simulink model "PumpSim"  (R2016b)
settings: Solver=VariableStepAuto  StartTime=0.0  StopTime=10.0  RelTol=1e-3
values from neighbouring files (symbols this model uses):
  A = pi*(0.00635)^2    (= 0.000126676869774)    [PumpParam.m]
  g = 9.8    [MotorParam.m]    (also in PumpParam.m)
  h = 0.5    [PumpParam.m]
  J = 0.02    [MotorParam.m]    (also in PumpParam.m)
  Kf = 0.2    [MotorParam.m]    (also in PumpParam.m)
  Km = 1    [MotorParam.m]    (also in PumpParam.m)
  L = 0.5    [MotorParam.m]    (also in PumpParam.m)
  M_amount = 10    [PumpParam.m]
  M_min = 3.75    [PumpParam.m]
  R = 2.0    (= 2)    [MotorParam.m]    (also in PumpParam.m)
  rho = 1    [PumpParam.m]
  T_fluid = 20    [PumpParam.m]
  T_fluidmin = 25    [PumpParam.m]
  v_pump = 5    [PumpParam.m]
libraries: simulink x3
settings Model: Creator=curtm  LastModifiedBy=curtm

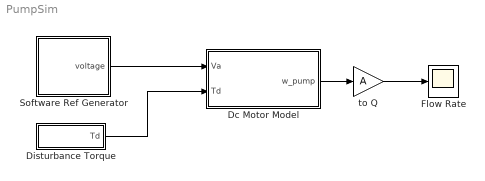
== system PumpSim ==
  Dc Motor Model : Subsystem
  Disturbance Torque : Subsystem
  Flow Rate : Scope
  Software Ref Generator : Subsystem
  to Q : Gain  Gain=A
  wires:
  Disturbance Torque/1(Td) -> Dc Motor Model/2(Td)
  Dc Motor Model/1(w_pump) -> to Q/1
  Software Ref Generator/1(voltage) -> Dc Motor Model/1(Va)
  to Q/1 -> Flow Rate/1

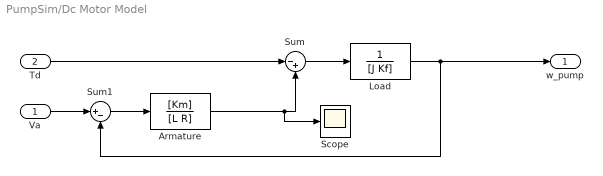
== system PumpSim/Dc Motor Model ==
  Va : Inport
  Td : Inport  Port=2
  Armature : TransferFcn  Numerator=[Km]  Denominator=[L R]
  Load : TransferFcn  Denominator=[J Kf]
  Scope : Scope
  Sum : Sum  Inputs=|-+
  Sum1 : Sum  Inputs=|+-
  w_pump : Outport
  wires:
  Va/1 -> Sum1/1
  Sum1/1 -> Armature/1
  Armature/1 -> Scope/1, Sum/2
  Td/1 -> Sum/1
  Load/1 -> w_pump/1, Sum1/2
  Sum/1 -> Load/1

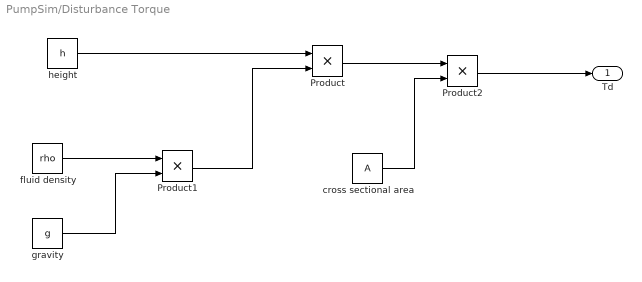
== system PumpSim/Disturbance Torque ==
  Product : Product
  Product1 : Product
  Product2 : Product
  cross sectional area : Constant  Value=A
  fluid density : Constant  Value=rho
  gravity : Constant  Value=g
  height : Constant  Value=h
  Td : Outport
  wires:
  Product/1 -> Product2/1
  Product1/1 -> Product/2
  height/1 -> Product/1
  fluid density/1 -> Product1/1
  gravity/1 -> Product1/2
  cross sectional area/1 -> Product2/2
  Product2/1 -> Td/1

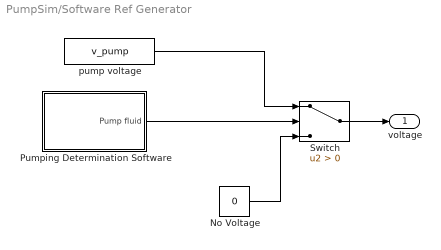
== system PumpSim/Software Ref Generator ==
  No Voltage : Constant  Value=0
  Pumping Determination Software : Subsystem
  Switch : Switch  Criteria=u2 > Threshold
  pump voltage : Constant  Value=v_pump
  voltage : Outport
  wires:
  Switch/1 -> voltage/1
  pump voltage/1 -> Switch/1
  No Voltage/1 -> Switch/3
  Pumping Determination Software/1(Pump fluid) -> Switch/2

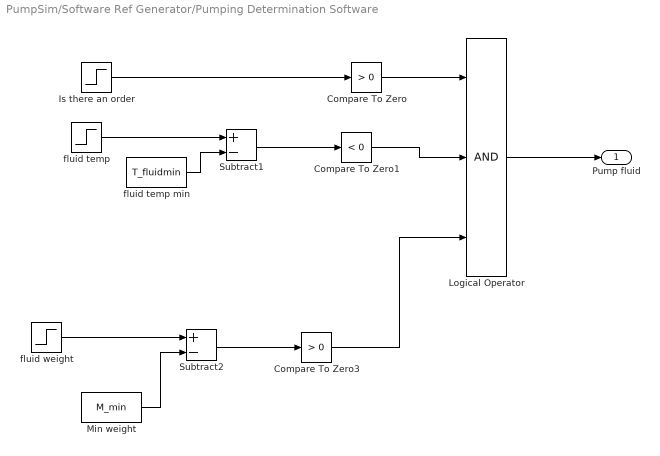
== system PumpSim/Software Ref Generator/Pumping Determination Software ==
  Compare To Zero : simulink/Logic and Bit Operations/Compare To Zero  relop=>  OutDataTypeStr=boolean
  Compare To Zero1 : simulink/Logic and Bit Operations/Compare To Zero  relop=<  OutDataTypeStr=boolean
  Compare To Zero3 : simulink/Logic and Bit Operations/Compare To Zero  relop=>  OutDataTypeStr=boolean
  "Is there an order " : Step  Time=0  SampleTime=0
  Logical Operator : Logic  Inputs=3  AllPortsSameDT=off  OutDataTypeStr=boolean
  Min weight : Constant  Value=M_min
  Subtract1 : Sum  Inputs=+-
  Subtract2 : Sum  Inputs=+-
  fluid temp : Step  Time=0  After=T_fluid  SampleTime=0
  fluid temp min : Constant  Value=T_fluidmin
  fluid weight : Step  Time=0  After=M_amount  SampleTime=0
  Pump fluid : Outport
  wires:
  Compare To Zero/1 -> Logical Operator/1
  "Is there an order "/1 -> Compare To Zero/1
  Logical Operator/1 -> Pump fluid/1
  Compare To Zero1/1 -> Logical Operator/2
  fluid temp/1 -> Subtract1/1
  Subtract1/1 -> Compare To Zero1/1
  fluid temp min/1 -> Subtract1/2
  Compare To Zero3/1 -> Logical Operator/3
  fluid weight/1 -> Subtract2/1
  Subtract2/1 -> Compare To Zero3/1
  Min weight/1 -> Subtract2/2
